simulink model "multirateTemplate"  (R2017b)
settings: Solver=VariableStepAuto  StartTime=0.0  StopTime=inf  RelTol=1e-3
PreLoadFcn:
  | % ROS setup
  | rosshutdown;
  | ipAddr = '';
  | rosinit(ipAddr)
  | 
  | % Sample times
  | sampleTimeSlow = 1;
  | sampleTimeFast = 0.2;
  | 
  | % Control parameters
  | ctrlParam1 = 2;
  | ctrlParam2 = 3.5;
undefined symbols (not defined in the file): X, Y
libraries: robotlib x4
settings Model: Creator=scastro  LastModifiedBy=scastro

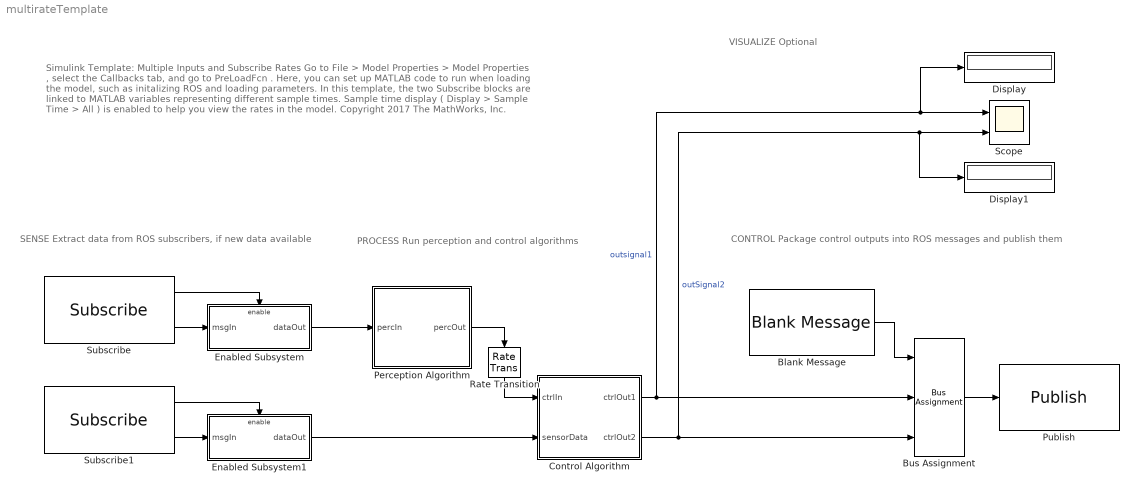
== system multirateTemplate ==
  note: PROCESS
      | Run perception and control algorithms
  note: SENSE
      | Extract data from ROS subscribers, if new data available
  note: VISUALIZE
      | Optional
  note: CONTROL
      | Package control outputs into ROS messages and publish them
  note: Simulink Template:
      | Multiple Inputs and Subscribe Rates
      |
      | Go to File > Model Properties > Model Properties , select the Callbacks tab, and go to PreLoadFcn .
      | Here, you can set up MATLAB code to run when loading the model, such as initalizing ROS and loading parameters.
      |
      | In this template, the two Subscribe blocks are linked to MATLAB variables representing different sample times.
      | Sample time display ( Display > Sample Time > All ) is enabled to help you view the rates in the model.
      |
      | Copyright 2017 The MathWorks, Inc.
  Blank Message : robotlib/Blank Message  SourceLibraryInfo=This block requires Robotics System Toolbox  messageType=geometry_msgs/Point  SampleTime=inf
      settings: SourceProductBaseCode=RO
  Bus Assignment : BusAssignment  AssignedSignals=X,Y
  Control Algorithm : Subsystem
  Display : Display
  Display1 : Display
  Enabled Subsystem : Subsystem  TreatAsAtomicUnit=on
  Enabled Subsystem1 : Subsystem  TreatAsAtomicUnit=on
  Perception Algorithm : Subsystem
  Publish : robotlib/Publish  SourceLibraryInfo=This block requires Robotics System Toolbox  topicSource=Specify your own  topic=/my_pub_topic  messageType=geometry_msgs/Point  messageQueueLength=1
      settings: SourceProductBaseCode=RO
  Rate Transition : RateTransition
  Scope : Scope  NumInputPorts=2
  Subscribe : robotlib/Subscribe  SourceLibraryInfo=This block requires Robotics System Toolbox  topicSource=Select from ROS network  topic=/my_sub_topic_1  messageType=geometry_msgs/Point  sampleTime=-1  messageQueueLength=1
      settings: SourceProductBaseCode=RO
  Subscribe1 : robotlib/Subscribe  SourceLibraryInfo=This block requires Robotics System Toolbox  topicSource=Select from ROS network  topic=/my_sub_topic_2  messageType=geometry_msgs/Point  sampleTime=-1  messageQueueLength=1
      settings: SourceProductBaseCode=RO
  wires:
  Enabled Subsystem/1(dataOut) -> Perception Algorithm/1(percIn)
  Subscribe/2 -> Enabled Subsystem/1(msgIn)
  Subscribe/1 -> Enabled Subsystem/Enable
  Bus Assignment/1 -> Publish/1
  Blank Message/1 -> Bus Assignment/1
  Perception Algorithm/1(percOut) -> Rate Transition/1
  Control Algorithm/1(ctrlOut1) -> Display/1, Scope/1, Bus Assignment/2  "outsignal1"
  Control Algorithm/2(ctrlOut2) -> Display1/1, Scope/2, Bus Assignment/3  "outSignal2"
  Subscribe1/1 -> Enabled Subsystem1/Enable
  Subscribe1/2 -> Enabled Subsystem1/1(msgIn)
  Enabled Subsystem1/1(dataOut) -> Control Algorithm/2(sensorData)
  Rate Transition/1 -> Control Algorithm/1(ctrlIn)

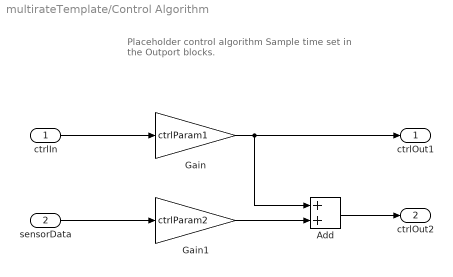
== system multirateTemplate/Control Algorithm ==
  note: Placeholder control algorithm
      |
      | Sample time set in the Outport blocks.
  ctrlIn : Inport
  sensorData : Inport  Port=2
  Add : Sum
  Gain : Gain  Gain=ctrlParam1
  Gain1 : Gain  Gain=ctrlParam2
  ctrlOut1 : Outport  SampleTime=sampleTimeFast
      settings: AttributesFormatString=Sample time: %<SampleTime>
  ctrlOut2 : Outport  Port=2  SampleTime=sampleTimeFast
      settings: AttributesFormatString=Sample time: %<SampleTime>
  wires:
  ctrlIn/1 -> Gain/1
  Gain/1 -> Add/1, ctrlOut1/1
  Add/1 -> ctrlOut2/1
  sensorData/1 -> Gain1/1
  Gain1/1 -> Add/2

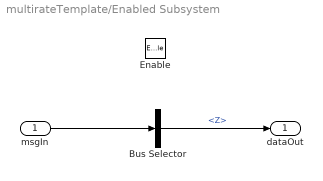
== system multirateTemplate/Enabled Subsystem ==
  msgIn : Inport
  Enable : EnablePort
  Bus Selector : BusSelector  OutputSignals=Z
  dataOut : Outport
  wires:
  msgIn/1 -> Bus Selector/1
  Bus Selector/1 -> dataOut/1  "<Z>"

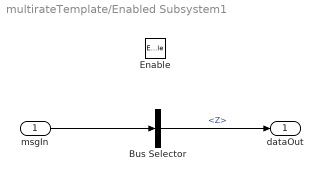
== system multirateTemplate/Enabled Subsystem1 ==
  msgIn : Inport
  Enable : EnablePort
  Bus Selector : BusSelector  OutputSignals=Z
  dataOut : Outport
  wires:
  msgIn/1 -> Bus Selector/1
  Bus Selector/1 -> dataOut/1  "<Z>"

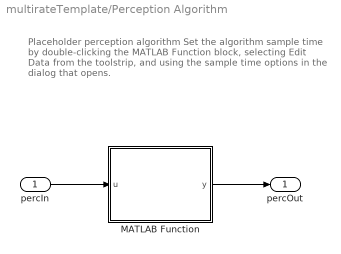
== system multirateTemplate/Perception Algorithm ==
  note: Placeholder perception algorithm
      |
      | Set the algorithm sample time by double-clicking the MATLAB Function block, selecting Edit Data from the toolstrip, and using the sample time options in the dialog that opens.
  percIn : Inport
  MATLAB Function : MATLAB Function  TreatAsAtomicUnit=on
  percOut : Outport
  wires:
  percIn/1 -> MATLAB Function/1(u)
  MATLAB Function/1(y) -> percOut/1

== matlab function multirateTemplate/Perception Algorithm/MATLAB Function ==
  settings: updateMethod=DISCRETE  sampleTime=sampleTimeSlow
  data: u input; y output
function y = myPerceptionFcn(u)

y = 2*u;
